simulink model "aero421_finalProjectSim_D"  (R2024a)
settings: Solver=FixedStepAuto  StartTime=0.0  StopTime=300  FixedStep=1  RelTol=1e-3
values from neighbouring files (symbols this model uses):
  CapOmegaDot0 = [0;0;0]    [aero421_finalProject_D.m]
  E0 = [phi0;theta0;psi0]    [aero421_finalProject.m]    (also in aero421_finalProject_D.m)
  E0_LVLH = [0;0;0]    [aero421_finalProject_D.m]
  Is = 1.2*eye(3)    [aero421_finalProject_D.m]
  Kd_rw = 2*zeta_rw*wn_rw*mehielSat.Jrw    [aero421_finalProject_D.m]
  Kp_rw = wn_rw^2*mehielSat.Jrw    [aero421_finalProject_D.m]
  Period = 2*pi*sqrt(norm(R_0)^3/mu)    [aero421_finalProject.m]    (also in aero421_finalProject_D.m)
  q0 = [n0;e0]    [aero421_finalProject.m]    (also in aero421_finalProject_D.m)
  q0_LVLH = [1;0;0;0]    [aero421_finalProject_D.m]
  state_0 = [R_0';V_0']    [aero421_finalProject.m]    (also in aero421_finalProject_D.m)
undefined symbols (not defined in the file or in its folder): mehielSat
settings Model: Creator=emehiel  LastModifiedBy=davey
settings SolverCC: AlgebraicLoopSolver=TrustRegion
settings DebuggingCC: UnconnectedInputMsg=warning  UnconnectedOutputMsg=warning  UnconnectedLineMsg=warning
settings ModelReferenceCC: EnableRefExpFcnMdlSchedulingChecks=on
settings RTWCC: GPUComputeCapability=3.5

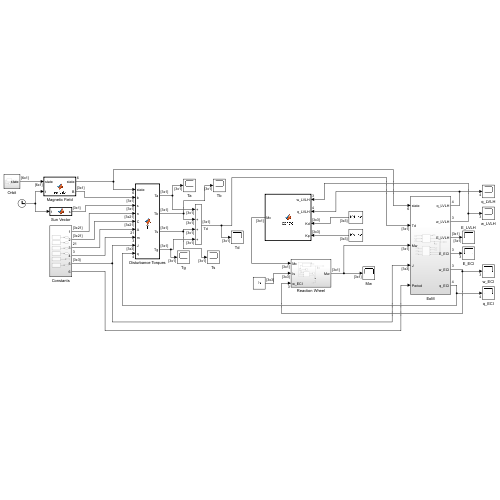
[thumbnail: Simulink's stored preview of the top-level diagram]
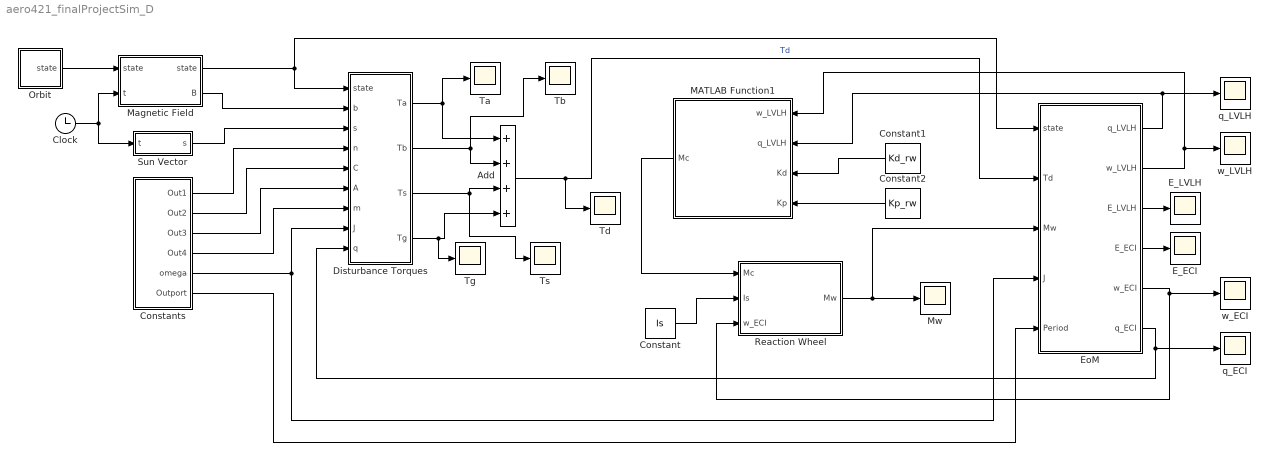
== system aero421_finalProjectSim_D ==
  Add : Sum  Inputs=++++
  Clock : Clock
  Constant : Constant  Value=Is
  Constant1 : Constant  Value=Kd_rw
  Constant2 : Constant  Value=Kp_rw
  Constants : Subsystem
  Disturbance Torques : MATLAB Function  TreatAsAtomicUnit=on
  E_ECI : Scope
  E_LVLH : Scope
  EoM : Subsystem
  MATLAB Function1 : MATLAB Function  TreatAsAtomicUnit=on
  Magnetic Field : MATLAB Function  TreatAsAtomicUnit=on
  Mw : Scope
  Orbit : Subsystem
  Reaction Wheel : Subsystem
  Sun Vector : MATLAB Function  TreatAsAtomicUnit=on
  Ta : Scope
  Tb : Scope
  Td : Scope
  Tg : Scope
  Ts : Scope
  q_ECI : Scope
  q_LVLH : Scope
  w_ECI : Scope
  w_LVLH : Scope
  wires:
  Magnetic Field/2(B) -> Disturbance Torques/2(b)
  Sun Vector/1(s) -> Disturbance Torques/3(s)
  Constants/1(Out1) -> Disturbance Torques/4(n)
  Constants/2(Out2) -> Disturbance Torques/5(C)
  Constants/3(Out3) -> Disturbance Torques/6(A)
  Constants/4(Out4) -> Disturbance Torques/7(m)
  Orbit/1(state) -> Magnetic Field/1("state ")
  Disturbance Torques/1(Ta) -> Add/1, Ta/1
  Disturbance Torques/2(Tb) -> Add/2, Tb/1
  Disturbance Torques/3(Ts) -> Ts/1, Add/3
  Magnetic Field/1(state) -> EoM/1(state), Disturbance Torques/1(state)
  Constants/5(omega) -> Disturbance Torques/8(J), EoM/4(J)
  EoM/2(w_LVLH) -> w_LVLH/1, MATLAB Function1/1(w_LVLH)
  EoM/1(q_LVLH) -> MATLAB Function1/2(q_LVLH), q_LVLH/1
  EoM/6(q_ECI) -> Disturbance Torques/9(q), q_ECI/1
  Constant1/1 -> MATLAB Function1/3(Kd)
  Constant2/1 -> MATLAB Function1/4(Kp)
  Clock/1 -> Sun Vector/1(t), Magnetic Field/2(t)
  Disturbance Torques/4(Tg) -> Tg/1, Add/4
  EoM/5(w_ECI) -> w_ECI/1, Reaction Wheel/3(w_ECI)
  MATLAB Function1/1(Mc) -> Reaction Wheel/1(Mc)
  Add/1 -> EoM/2(Td), Td/1  "Td"
  Reaction Wheel/1(Mw) -> EoM/3(Mw), Mw/1
  Constant/1 -> Reaction Wheel/2(Is)
  Constants/6(Outport) -> EoM/5(Period)
  EoM/4(E_ECI) -> E_ECI/1
  EoM/3(E_LVLH) -> E_LVLH/1

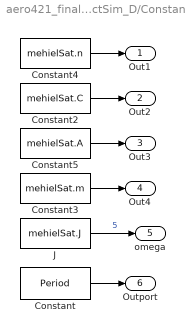
== system aero421_finalProjectSim_D/Constants ==
  Constant : Constant  Value=Period
  Constant2 : Constant  Value=mehielSat.C
  Constant3 : Constant  Value=mehielSat.m
  Constant4 : Constant  Value=mehielSat.n
  Constant5 : Constant  Value=mehielSat.A
  J : Constant  Value=mehielSat.J
  Out1 : Outport
  Out2 : Outport  Port=2
  Out3 : Outport  Port=3
  Out4 : Outport  Port=4
  omega : Outport  Port=5
  Outport : Outport  Port=6
  wires:
  J/1 -> omega/1  "5"
  Constant2/1 -> Out2/1
  Constant3/1 -> Out4/1
  Constant4/1 -> Out1/1
  Constant5/1 -> Out3/1
  Constant/1 -> Outport/1

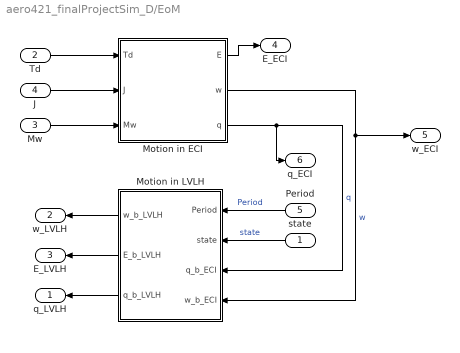
== system aero421_finalProjectSim_D/EoM ==
  state : Inport
  Td : Inport  Port=2
  Mw : Inport  Port=3
  J : Inport  Port=4
  Period : Inport  Port=5
  Motion in ECI : Subsystem
  Motion in LVLH : Subsystem
  q_LVLH : Outport
  w_LVLH : Outport  Port=2
  E_LVLH : Outport  Port=3
  E_ECI : Outport  Port=4
  w_ECI : Outport  Port=5
  q_ECI : Outport  Port=6
  wires:
  Motion in ECI/3(q) -> Motion in LVLH/3(q_b_ECI), q_ECI/1  "q"
  Motion in ECI/2(w) -> w_ECI/1, Motion in LVLH/4(w_b_ECI)  "w"
  state/1 -> Motion in LVLH/2("state ")  "state"
  Td/1 -> Motion in ECI/1(Td)
  Motion in LVLH/2(E_b_LVLH) -> E_LVLH/1
  Motion in ECI/1(E) -> E_ECI/1
  J/1 -> Motion in ECI/2(J)
  Motion in LVLH/1(w_b_LVLH) -> w_LVLH/1
  Motion in LVLH/3(q_b_LVLH) -> q_LVLH/1
  Period/1 -> Motion in LVLH/1(Period)  "Period"
  Mw/1 -> Motion in ECI/3(Mw)

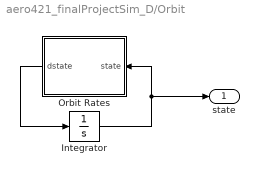
== system aero421_finalProjectSim_D/Orbit ==
  Integrator : Integrator  InitialCondition=state_0
  Orbit Rates : MATLAB Function  TreatAsAtomicUnit=on
  state : Outport
  wires:
  Integrator/1 -> Orbit Rates/1(state), state/1
  Orbit Rates/1(dstate) -> Integrator/1

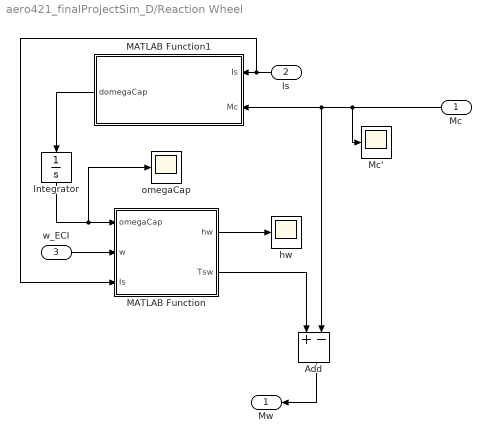
== system aero421_finalProjectSim_D/Reaction Wheel ==
  Mc : Inport
  Is : Inport  Port=2
  w_ECI : Inport  Port=3
  Add : Sum  Inputs=+-
  Integrator : Integrator  InitialCondition=CapOmegaDot0
  MATLAB Function : MATLAB Function  TreatAsAtomicUnit=on
  MATLAB Function1 : MATLAB Function  TreatAsAtomicUnit=on
  Mc' : Scope
  hw : Scope
  omegaCap : Scope
  Mw : Outport
  wires:
  Mc/1 -> Mc'/1, Add/2, MATLAB Function1/2(Mc)
  w_ECI/1 -> MATLAB Function/2(w)
  Add/1 -> Mw/1
  MATLAB Function/1(hw) -> hw/1
  MATLAB Function/2(Tsw) -> Add/1
  Is/1 -> MATLAB Function/3(Is), MATLAB Function1/1(Is)
  MATLAB Function1/1(domegaCap) -> Integrator/1
  Integrator/1 -> omegaCap/1, MATLAB Function/1(omegaCap)

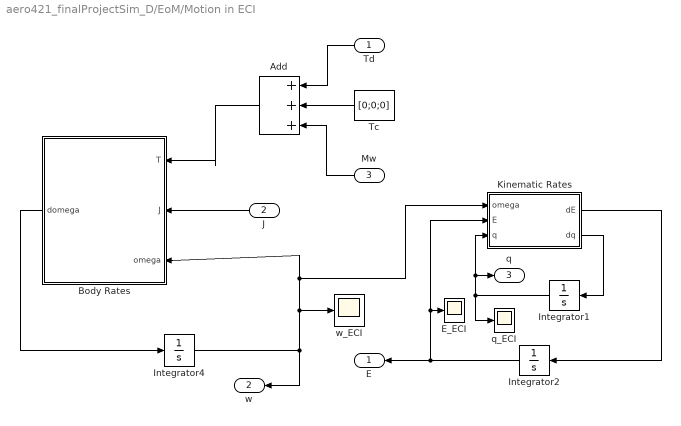
== system aero421_finalProjectSim_D/EoM/Motion in ECI ==
  Td : Inport
  J : Inport  Port=2
  Mw : Inport  Port=3
  Add : Sum  Inputs=+++
  Body Rates : MATLAB Function  TreatAsAtomicUnit=on
  E_ECI : Scope
  Integrator1 : Integrator  InitialCondition=q0
  Integrator2 : Integrator  InitialCondition=E0
  Integrator4 : Integrator  InitialCondition=mehielSat.w0
  Kinematic Rates : MATLAB Function  TreatAsAtomicUnit=on
  Tc : Constant  Value=[0;0;0]  OutDataTypeStr=Inherit: Inherit via back propagation
  q_ECI : Scope
  w_ECI : Scope
  E : Outport
  w : Outport  Port=2
  q : Outport  Port=3
  wires:
  Integrator1/1 -> q/1, Kinematic Rates/3(q), q_ECI/1
  Kinematic Rates/2(dq) -> Integrator1/1
  Kinematic Rates/1(dE) -> Integrator2/1
  Body Rates/1(domega) -> Integrator4/1
  J/1 -> Body Rates/2(J)
  Integrator2/1 -> E_ECI/1, Kinematic Rates/2(E), E/1
  Integrator4/1 -> w/1, w_ECI/1, Body Rates/3(omega), Kinematic Rates/1(omega)
  Td/1 -> Add/1
  Mw/1 -> Add/3
  Add/1 -> Body Rates/1(T)
  Tc/1 -> Add/2

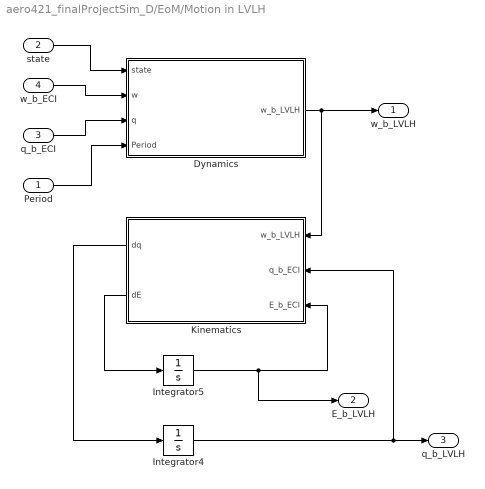
== system aero421_finalProjectSim_D/EoM/Motion in LVLH ==
  Period : Inport
  "state " : Inport  Port=2
  q_b_ECI : Inport  Port=3
  w_b_ECI : Inport  Port=4
  Dynamics : MATLAB Function  TreatAsAtomicUnit=on
  Integrator4 : Integrator  InitialCondition=q0_LVLH
  Integrator5 : Integrator  InitialCondition=E0_LVLH
  Kinematics : MATLAB Function  TreatAsAtomicUnit=on
  w_b_LVLH : Outport  VectorParamsAs1DForOutWhenUnconnected=off
  E_b_LVLH : Outport  Port=2  PortDimensions=[3 1]  VectorParamsAs1DForOutWhenUnconnected=off
  q_b_LVLH : Outport  Port=3  VectorParamsAs1DForOutWhenUnconnected=off
  wires:
  w_b_ECI/1 -> Dynamics/2(w)
  q_b_ECI/1 -> Dynamics/3(q)
  "state "/1 -> Dynamics/1(state)
  Dynamics/1(w_b_LVLH) -> w_b_LVLH/1, Kinematics/1(w_b_LVLH)
  Integrator4/1 -> Kinematics/2(q_b_ECI), q_b_LVLH/1
  Integrator5/1 -> Kinematics/3(E_b_ECI), E_b_LVLH/1
  Kinematics/1(dq) -> Integrator4/1
  Kinematics/2(dE) -> Integrator5/1
  Period/1 -> Dynamics/4(Period)

== matlab function aero421_finalProjectSim_D/EoM/Motion in LVLH/Dynamics ==
  data: state input; w input; q input; w_b_LVLH output; Period input
function w_b_LVLH = DynamicsLVLH(state, w, q, Period)

% Unpack State
r_ECI = state(1:3);
v_ECI = state(4:6);

% Unpack Quaternion
n = q(1);
e = q(2:4);

% Rotation Matrix, ECI to Body
C_B_ECI = (2*n^2-1)*eye(3) + 2 * (e*e') - 2*n*vect2cross(e);

% Angular Momentum, ECI w.r.t. LVLH
h_ECI_LVLH = cross(r_ECI,v_ECI);

% Angular Velocity, LVLH w.r.t. ECI
w_LVLH_ECI = C_B_ECI*(h_ECI_LVLH/norm(r_ECI)^2);

% Angular Velocity, Body w.r.t. ECI
w_b_LVLH = w - w_LVLH_ECI;

function ax = vect2cross(a)

ax = [0 -a(3) a(2); a(3) 0 -a(1); -a(2) a(1) 0];

end
end

== matlab function aero421_finalProjectSim_D/EoM/Motion in LVLH/Kinematics ==
  data: w_b_LVLH input; q_b_ECI input; dq output; E_b_ECI input; dE output
function [dq,dE] = KinematicsLVLH(w_b_LVLH, q_b_ECI, E_b_ECI)

% unpack quaternion

n = q_b_ECI(1);
e = q_b_ECI(2:4);

% compute the derivative of the quaternion components here

dn = -1/2 * e' * w_b_LVLH;
de =  1/2 * (n * eye(3) + vect2cross(e)) * w_b_LVLH;

dq = [dn; de];

% compute the derivative of the Euler Angle components here
phi   = E_b_ECI(1);
theta = E_b_ECI(2);

% Rotation from Body to LVLH
LBI = 1/cos(theta)*[cos(theta) sin(phi)*sin(theta)  cos(phi)*sin(theta);
                     0         cos(phi)*cos(theta) -sin(phi)*cos(theta);
                     0              sin(phi)             cos(phi)     ];

dE = LBI*w_b_LVLH;

function ax = vect2cross(a)

ax = [0 -a(3) a(2); a(3) 0 -a(1); -a(2) a(1) 0];

end
end

== matlab function aero421_finalProjectSim_D/Reaction Wheel/MATLAB Function1 ==
  data: Is input; domegaCap output; Mc input
function domegaCap = omegaCappa(Is,Mc)

domegaCap = Is\Mc;

== matlab function aero421_finalProjectSim_D/Magnetic Field ==
  data: state output; state input; t input; B output
function [state,B] = earthB(state,t)

i = t;

sec = rem(i,60);
i = (i - sec) / 60;

min = rem(i,60);
i = (i - min) / 60;

hrs = rem(i,24);
i = (i - hrs) / 24;

day = rem(i,31)+20;
i = (i - (day-1)) / 31;

mon = rem(i,12)+3;
i = (i - (mon-1)) / 12;

yrs = i + 2024;

time = [yrs mon day hrs min sec];

% initialize aerospace toolbox functions into simulink
coder.extrinsic("eci2ecef")
coder.extrinsic("ecef2eci")

% Initialize r vector in simulink for type setting
r = zeros(3,1);

% convert current r from eci to ecef
r = eci2ecef(time,state(1:3)); % km
r = r * 1000; % m
r_= norm(r);  % norm of r calculated for effeciency

a =   6371.2; % km
a = a * 1000; %  m

g11 = -1450.9;  % nT
h11 =  4652.5;  % nT
g01 =-29404.8;  % nT

g11 = g11 * 10^-9;  % T
h11 = h11 * 10^-9;  % T
g01 = g01 * 10^-9;  % T

m = a^3 * [g11;h11;g01]; % m^3*T

B = ((3 * m'*r) * r - r_^2 * m) / r_^5; % T
B = ecef2eci(time,B); % Convert B vector into ECI

end

== matlab function aero421_finalProjectSim_D/Disturbance Torques ==
  data: state input; b input; s input; n input; C input; A input; m input; J input; Ta output; Tb output; Ts output; Tg output; q input
function [Ta,Tb,Ts,Tg] = T(state,b,s,n,C,A,m,J,q)

% s,b,state input in ECI
% n,C,m,J input in Body
% A input in scalar

% T output needs to be in body

% Pull out R and V vectors from state vector
R = state(1:3);
V = state(4:6);

% unpack quaternion
eta = q(1);
eps = q(2:4);

% Use euler angles to calculate rotation matrix from ECI to body
C_ECI_B = ( 2 * eta^2 - 1) * eye(3) + (2 * eps * eps') - 2 * eta * vect2cross(eps);

% Use rotation matrix to get ECI vectors into body
rb = C_ECI_B*R*1000; % R in meters
V  = C_ECI_B*V*1000; % V in m/s
s  = C_ECI_B*s;      % Sun direction vector
b  = C_ECI_B*b;      % Earth's magnetic field

%% Atmospheric Drag Torque, Ta

% Atmospherice Drag Torgue, preallocated
Ta = zeros(3,1);

% s/c velocity
v = norm(V); % speed, m/s
vhat = V/v; % velocity as unit vector, m/s 

% constants
rhoA = 1.644608e-14; % Atmospheric Density, kg/m^3
Cd = 2.5; % Coefficient of Drag, unitless

for i = 1:21
    if dot(n(:,i),vhat) > 0
        Cp = C(:,i); % center of pressure, m
        Fa = -1/2 * rhoA * v^2 * Cd * A(i) * vhat; % Drag Force, N
        Ta = Ta + cross(Cp,Fa); % Atmospheric Drag Torque, N*m
    end
end

%% Magnetic Field Torque, Tb
Tb = cross(m,b); % N*m

%% SRP Torque, Ts

% Preallocated SRP Torque Vector
Ts = zeros(3,1);

% constants 
p = 4.5e-6; % Solar Pressure in Earth Orbit, in N/m^2

for i = 1:21
    if dot(n(:,i),s) > 0
        Cp = C(:,i);
        Fa = -p * s * A(i); % SRP force on s/c, N
        Ts = Ts + cross(Cp,Fa); % SRP Torque, N*m
    end
end

%% Gravity Gradient Torque, Tg

% constants
mu = 3.98600e14; % gravitational parameter kg^2/m^3

rx = vect2cross(rb); % vector cross of position vector, m

Tg = ((3 * mu) / norm(rb)^5) * rx * J * rb; % Gravity Gradient Torque, N*m

%% Sub Functions
function ax = vect2cross(a)

ax = [0 -a(3) a(2); a(3) 0 -a(1); -a(2) a(1) 0];

end

function [C] = basicrot(a,theta)

if a == 1
    C = [1 0 0 ; 0 cosd(theta) sind(theta); 0 -sind(theta) cosd(theta)];
elseif a == 2
    C = [cosd(theta) 0 -sind(theta); 0 1 0; sind(theta) 0 cosd(theta)];
elseif a == 3
    C = [cosd(theta) sind(theta) 0; -sind(theta) cosd(theta) 0; 0 0 1];
end
end


end

== matlab function aero421_finalProjectSim_D/Orbit/Orbit Rates ==
  data: dstate output; state input
function dstate  = orbitRates(state)

mu = 398600; % gravitational parameter, in km

x = state(1);
y = state(2);
z = state(3);
dx = state(4);
dy = state(5);
dz = state(6);

r = norm([x y z]);

ddx = -mu * x / r^3;
ddy = -mu * y / r^3;
ddz = -mu * z / r^3;

dstate = [dx;dy;dz;ddx;ddy;ddz];

== matlab function aero421_finalProjectSim_D/Reaction Wheel/MATLAB Function ==
  data: omegaCap input; w input; hw output; Is input; Tsw output
function [hw,Tsw] = gyrocoup(omegaCap,w,Is)

hw = Is*omegaCap;

Tsw = -cross(w,hw);

== matlab function aero421_finalProjectSim_D/MATLAB Function1 ==
  data: w_LVLH input; q_LVLH input; Kd input; Kp input; Mc output
function Mc  = control(w_LVLH,q_LVLH,Kd,Kp)

% Quaternion Control
qc = [1;0;0;0];

% Quaternion Error
qe = quatMult(quatConj(qc),q_LVLH);

% Epsilon Error
epsilonError = qe(2:4);

% Control Torque
Mc = Kp*epsilonError + Kd*w_LVLH;

function q_star = quatConj(q)
    q_star = [q(4);-q(1:3)];
end
function qAns = quatMult(q1,q2)
% Quaternion Multiplication
% Inputs: Two quaternions in form [n;e]

w1 = q1(1);
x1 = q1(2);
y1 = q1(3);
z1 = q1(4);

w2 = q2(1);
x2 = q2(2);
y2 = q2(3);
z2 = q2(4);

qAns = [(w1*w2 - x1*x2 - y1*y2 - z1*z2); ...
        (w1*x2 + x1*w2 + y1*z2 - z1*y2); ...
        (w1*y2 - x1*z2 + y1*w2 + z1*x2); ...
        (w1*z2 + x1*y2 - y1*x2 + z1*w2)];
end
end

== matlab function aero421_finalProjectSim_D/EoM/Motion in ECI/Body Rates ==
  data: T input; J input; omega input; domega output
function domega = dynamics(T, J, omega)

% Using the Euler Equations
domega = J\(T-cross(omega,J*omega));

== matlab function aero421_finalProjectSim_D/Sun Vector ==
  data: t input; s output
function s = sunVector(t)

% https://www.mathworks.com/matlabcentral/fileexchange/114710-investigation-of-the-sun-direction-vector-in-eci

JD = 2.4603895e+06 + (t/86400);

T_UT1= (JD - 2451545)/36525;
% The mean longitude of the sun
delta_M_Sun= 280.460 + 36000.770*T_UT1;
T_TDB= T_UT1;
% The mean anomaly of the sun
M_Sun= 357.5277233 + 35999.05034*T_TDB;
% The ecliptic longitude of the sun
delta_ecliptic= delta_M_Sun + 1.914666471*sind(M_Sun) + 0.019994643*sin(2*M_Sun);
% The linear model of the ecliptic of the sun
E= 23.439291 - 0.0130042*T_TDB;
% The unit sun vector is given in the ECI frame
s = [cosd(delta_ecliptic); sind(delta_ecliptic).*cosd(E); sind(delta_ecliptic).*sind(E)];

== matlab function aero421_finalProjectSim_D/EoM/Motion in ECI/Kinematic Rates ==
  data: dE output; omega input; E input; q input; dq output
function [dE,dq] = kinematics(omega, E, q)

% The spacecraft initial attitude is such that it is aligned with F_LVLH
% Compute initial quaternion and EULER angles relating Fb and Feci

% unpack quaternion
n = q(1);
e = q(2:4);

% derivative of quaternion
dn = -1/2 * e' * omega;
de =  1/2 * (n * eye(3) + vect2cross(e)) * omega;
dq = [dn;de];

% euler angles
phi   = E(1);
theta = E(2);

% Rotation from ECI to Body
LBI = 1/cos(theta)*[cos(theta) sin(phi)*sin(theta)  cos(phi)*sin(theta);
                     0         cos(phi)*cos(theta) -sin(phi)*cos(theta);
                     0              sin(phi)             cos(phi)     ];
dE = LBI*omega;

function ax = vect2cross(a)

ax = [0 -a(3) a(2); a(3) 0 -a(1); -a(2) a(1) 0];

end

end
